simulink model "dpsk_transmit"  (R2022a)
settings: Solver=FixedStepDiscrete  StartTime=0.0  StopTime=1  FixedStep=0.01  RelTol=1e-3
model workspace (MAT data in the model file):
  imageBits = [0 1 0 1]
  rrc = [-0.98185278585 -0.897032467763 -0.806551534552 -0.710399295652 -0.608574997182 -0.501087965073 -0.387957728719 -0.269214124696 -0.144897380152 -0.0150581754827 0.120242314009 0.260932397749 ... (160 elements, 1x160)]
settings Model: Creator=luoch  LastModifiedBy=luoch
settings DataIOCC: SaveOutput=off  SignalLogging=off
settings ModelReferenceCC: EnableRefExpFcnMdlSchedulingChecks=off
settings RTWCC: Description=Generic Real-Time Target  GPUComputeCapability=5.0
settings ConfigComp: CovBoundaryAbsTol=1.0e-5

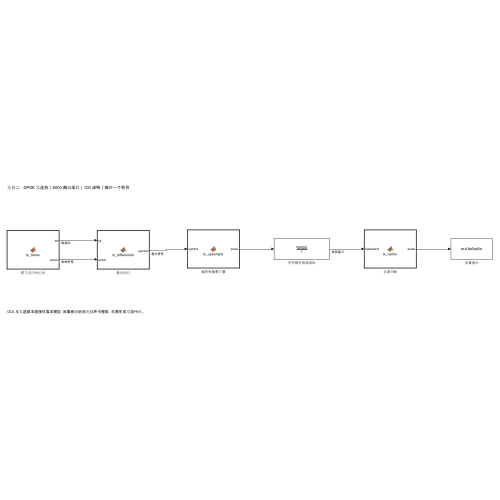
[thumbnail: Simulink's stored preview of the top-level diagram]
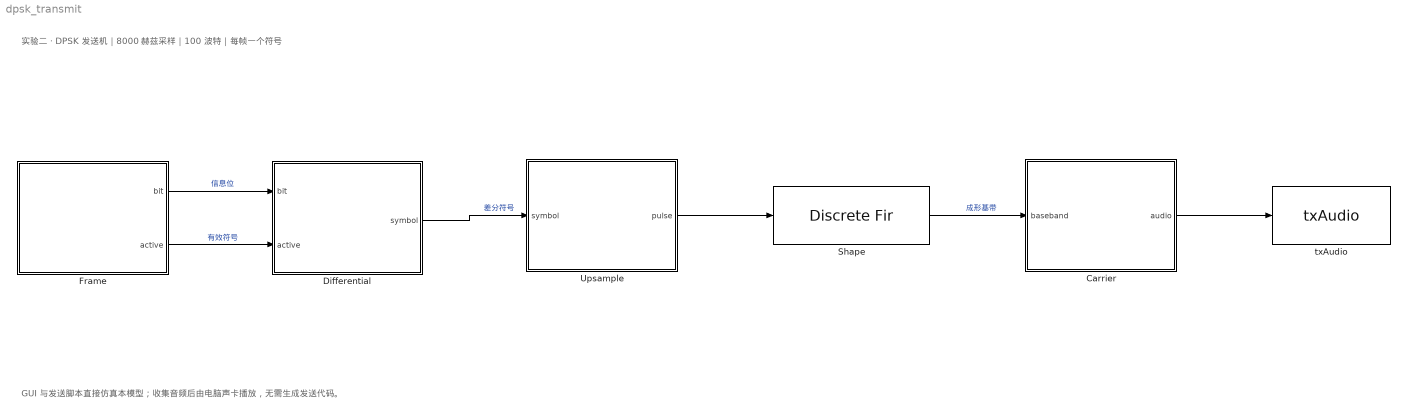
== system dpsk_transmit ==
  note: 实验二 · DPSK 发送机｜8000 赫兹采样｜100 波特｜每帧一个符号
  note: GUI 与发送脚本直接仿真本模型；收集音频后由电脑声卡播放，无需生成发送代码。
  Carrier : MATLAB Function  TreatAsAtomicUnit=on
      settings: AttributesFormatString=载波调制
  Differential : MATLAB Function  TreatAsAtomicUnit=on
      settings: AttributesFormatString=差分编码
  Frame : MATLAB Function  TreatAsAtomicUnit=on
      settings: AttributesFormatString=前导与图片组帧
  Shape : DiscreteFir  Coefficients=rrc  InputProcessing=Columns as channels (frame based)
      settings: AttributesFormatString=平方根升余弦成形
  Upsample : MATLAB Function  TreatAsAtomicUnit=on
      settings: AttributesFormatString=每符号插零扩展
  txAudio : ToWorkspace  VariableName=txAudio  SampleTime=-1
      settings: AttributesFormatString=仿真音频
  wires:
  Frame/1(bit) -> Differential/1(bit)  "信息位"
  Frame/2(active) -> Differential/2(active)  "有效符号"
  Differential/1(symbol) -> Upsample/1(symbol)  "差分符号"
  Upsample/1(pulse) -> Shape/1
  Shape/1 -> Carrier/1(baseband)  "成形基带"
  Carrier/1(audio) -> txAudio/1

== matlab function dpsk_transmit/Frame ==
  settings: updateMethod=DISCRETE  sampleTime=0.01
  data: bit output; active output; imageBits parameter
function [bit,active]=tx_frame(imageBits)
%#codegen
% 前导、交替段、首尾 m 序列、图片比特及尾部保护，均在模型内产生。
persistent index
if isempty(index),index=1;end
mseq=[1 0 0 1 1 0 1 0 1 1 1 1 0 0 0];alternate=[0 1 0 1 0 1 0 1];
L=numel(imageBits);active=index<=56+L+80;bit=0;
if index>=19 && index<27,bit=alternate(index-18);
elseif index>=27 && index<42,bit=mseq(index-26);
elseif index>=42 && index<42+L,bit=imageBits(index-41);
elseif index>=42+L && index<57+L,bit=mseq(index-41-L);
end
index=index+1;
end

== matlab function dpsk_transmit/Upsample ==
  settings: updateMethod=DISCRETE  sampleTime=0.01
  data: symbol input; pulse output
function pulse=tx_upsample(symbol)
%#codegen
% 每符号 80 点，首点放置脉冲，其余补零。
pulse=zeros(80,1);pulse(1)=symbol;
end

== matlab function dpsk_transmit/Carrier ==
  settings: updateMethod=DISCRETE  sampleTime=0.01
  data: baseband input; audio output
function audio=tx_carrier(baseband)
%#codegen
% 成形基带乘以连续的 1000 赫兹正弦载波。
persistent sample
if isempty(sample),sample=0;end
audio=baseband.*sin(2*pi*1000*(sample+(0:79)')/8000);sample=sample+80;
end

== matlab function dpsk_transmit/Differential ==
  settings: updateMethod=DISCRETE  sampleTime=0.01
  data: bit input; symbol output; active input
function symbol=tx_differential(bit,active)
%#codegen
% 当前相位由信息位与上一相位异或得到；冲洗滤波器时输出零。
persistent state
if isempty(state),state=false;end
symbol=0;
if active,state=xor(bit~=0,state);symbol=1-2*double(state);end
end
